simulink model "mdex_data_type_conversion_rwv_and_si"  (R2013b)
settings: Solver=FixedStepDiscrete  StartTime=0.0  StopTime=10.0  FixedStep=1  RelTol=1e-3
settings Model: Creator=The MathWorks Inc.  LastModifiedBy=Think79
settings DataIOCC: SignalLoggingSaveFormat=ModelDataLogs
settings OptimizationCC: ExpressionDepthLimit=2147483647
settings DebuggingCC: FcnCallInpInsideContextMsg=UseLocalSettings  StateNameClashWarn=warning
settings RTWCC: ProcessScript=grt_make_rtw_hook
settings GRTTargetCC: CombineOutputUpdateFcns=off  GRTInterface=on

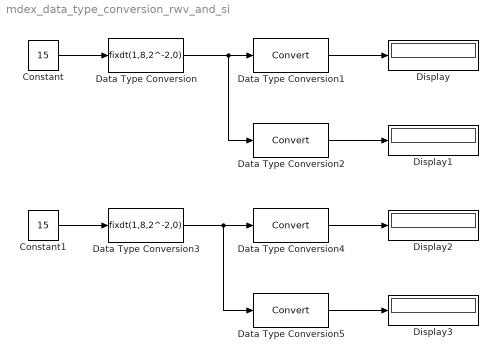
== system mdex_data_type_conversion_rwv_and_si ==
  Constant : Constant  Value=15
  Constant1 : Constant  Value=15
  Data Type Conversion : DataTypeConversion  OutDataTypeStr=fixdt(1,8,2^-2,0)
  Data Type Conversion1 : DataTypeConversion
  Data Type Conversion2 : DataTypeConversion  ConvertRealWorld=Stored Integer (SI)
  Data Type Conversion3 : DataTypeConversion  OutDataTypeStr=fixdt(1,8,2^-2,0)  ConvertRealWorld=Stored Integer (SI)
  Data Type Conversion4 : DataTypeConversion
  Data Type Conversion5 : DataTypeConversion  ConvertRealWorld=Stored Integer (SI)
  Display{,1..3} (4 alike) : Display
  wires:
  Constant/1 -> Data Type Conversion/1
  Data Type Conversion/1 -> Data Type Conversion1/1, Data Type Conversion2/1
  Data Type Conversion1/1 -> Display/1
  Data Type Conversion2/1 -> Display1/1
  Constant1/1 -> Data Type Conversion3/1
  Data Type Conversion3/1 -> Data Type Conversion4/1, Data Type Conversion5/1
  Data Type Conversion4/1 -> Display2/1
  Data Type Conversion5/1 -> Display3/1
